simulink library "dali_library"  (Simulink 7.4)
settings: Solver=ode45  StartTime=0.0  StopTime=10.0  RelTol=1e-3
libraries: dali_library x65, xbsIndex_r4 x43, gavrt_library x10, casper_library x1
settings Model: Creator=rprimian  LastModifiedBy=rprimian

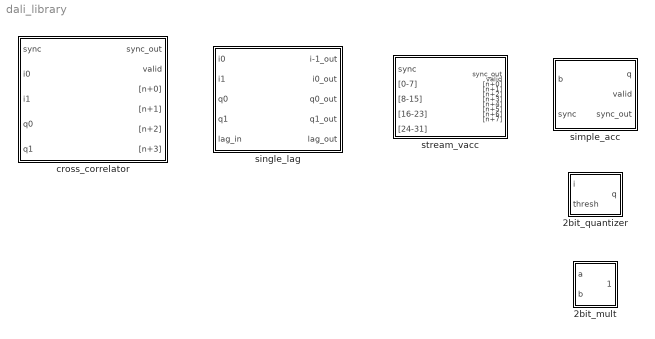
== system dali_library ==
  2bit_mult : Subsystem
      mask Type: 2bit_mult
      mask Description: Implements a special 2-bit multiplier in regular slices. The states represent a symmetric binary encoding where 0, 1, -1, -2 are small-positive, large-positive, small-negative, and large-negative respectively. This is compatible with the 2-bit quantizer
      mask Display:
      | port_label('input', 1, 'a');
      | port_label('input', 2, 'b');
      | port_label('output', 1, '(ab)');
  2bit_quantizer : Subsystem
      mask Type: 2bit_quantizer
      mask Description: Quantizes inputs to a special 2-bit binary encoding using a dynamically set threshold value.
  cross_correlator : Subsystem  mask(cross_correlator){total_lags=5, n_inputs=1, use_2bit=off, input_bit_width=8, input_bin_pt=7, specify_data_type=off, output_bit_width=16, output_bin_pt=14, quantization=Truncate, overflow=Wrap, specify_mult=off, mult_spec=Behavioral, specify_add=off, add_spec=Fabric, mult_delay=3, add_delay=2, single_output=off}
      mask prompts: total_lags "Total Lags Centered at Zero: (2^?)"; n_inputs "Number of Simultaneous Inputs: (2^?)"; use_2bit "Use special 2-bit binary encoding"; input_bit_width "Input Bit Width:"; input_bin_pt "Input Binary Point:"; specify_data_type "Specify output data type"; output_bit_width "Output Bit Width:"; output_bin_pt "Output Binary Point:"; quantization "Quantization Behavior:"; overflow "Overflow Behavior"; specify_mult "Specify multiplier use (behavioural HDL if not specified)"; mult_spec "Multiplier specification:"; specify_add "Specify adder use (behavioural HDL if not specified)"; add_spec "Adder specification:"; mult_delay "Mult Latency:"; add_delay "Add Latency:"; single_output "Provide single output stream"
      mask help: This time-domain cross correlator accepts two real time-series and outputs the cross-correlation function for the given set of lags. The output is accumulated so that for every two input samples there is exactly one output sample.
      mask init:
      | cross_correlator_init(gcb,...
      |     'total_lags', total_lags,...
      |     'n_inputs', n_inputs,...
      |     'use_2bit', use_2bit,...
      |     'input_bit_width', input_bit_width,...
      |     'input_bin_pt', input_bin_pt,...
      |     'specify_data_type', specify_data_type,...
      |     'output_bit_width', output_bit_width,...
      |     'output_bin_pt', output_bin_pt,...
      |     'quantization', quantization,...
      |     'overflow', overflow,...
      |     'specify_mult', specify_mult,...
      |     'mult_spec', mult_spec,...
      |     'specify_add', specify_add,...
      |     'add_spec', add_spec,...
      |     'mult_delay', mult_delay,...
      |     'add_delay', add_delay,...
      |     'single_output', single_output);
      settings: AttributesFormatString=|
      | 32 lags, Demux: 2, Outputs: 4
      | 8_7=>16_14, Truncate, Wrap
      |  Mult: Behavioral, Add: Fabric
      mask StyleString: edit,edit,checkbox,edit,edit,checkbox,edit,edit,popup(Truncate|Round (unbiased: +/- Inf)|Round (unbiased: Even Values)),popup(Wrap|Saturate|Flag as error),checkbox,popup(Behavioral|Core|Embedded),checkbox,popup(Fabric|DSP48),edit,edit,checkbox
      mask CallbackString:
      | ||use_2bit = get_param(gcb,'use_2bit');
      | enables = get_param(gcb, 'MaskEnables');
      | if( strcmp(use_2bit,'on')),
      |     enables{4} = 'off';
      |     enables{5} = 'off';
      | else
      |     enables{4} = 'on';
      |     enables{5} = 'on';
      | end
      | set_param(gcb, 'MaskEnables', enables);
      | |||specify_data_type = get_param(gcb,'specify_data_type');
      | enables = get_param(gcb, 'MaskEnables');
      | if( strcmp(specify_data_type,'off')),
      |     enables{7} = 'off';
      |     enables{8} = 'off';
      |     enables{9} = 'off';
      |     enables{10} = 'off';
      | else
      |     enables{7} = 'on';
      |     enables{8} = 'on';
      |     enables{9} = 'on';
      |     enables{10} = 'on';
      | end
      | set_param(gcb, 'MaskEnables', enables);
      | |||||specify_mult = get_param(gcb,'specify_mult');
      | enables = get_param(gcb, 'MaskEnables');
      | if( strcmp(specify_mult,'off')),
      |     enables{12} = 'off';
      | else
      |     enables{12} = 'on';
      | end
      | set_param(gcb, 'MaskEnables', enables);
      | ||specify_add = get_param(gcb,'specify_add');
      | enables = get_param(gcb, 'MaskEnables');
      | if( strcmp(specify_add,'off')),
      |     enables{14} = 'off';
      | else
      |     enables{14} = 'on';
      | end
      | set_param(gcb, 'MaskEnables', enables);
      | ||||
      mask TabNameString: Basic,Basic,Input,Input,Input,Output,Output,Output,Output,Output,Implementation,Implementation,Implementation,Implementation,Implementation,Implementation,Basic
  simple_acc : Subsystem  mask(simple_acc){samples=2, bit_width=16, bin_pt=14, quantization=Truncate, overflow=Flag as error, specify_add=off, add_spec=Fabric}
      mask prompts: samples "Samples to Accumulate: (2^?)"; bit_width "Output Bit Width:"; bin_pt "Output Binary Point:"; quantization "Quantization Behavior:"; overflow "Overflow Behavior:"; specify_add "Specify adder use (behavioural HDL if not specified)"; add_spec "Adder Specification:"
      mask help: This block accumulates a single stream of data for 2^n samples at a time. The partial sums are full every 2^n clocks and are synced to the falling edge of the sync_out port.
      mask init:
      | set_param([gcb, '/AddSub'], 'Quantization', quantization);
      | set_param([gcb, '/AddSub'], 'Overflow', overflow);
      | if strcmp(specify_add, 'on')
      |     set_param([gcb, '/AddSub'], 'Use_Behavioral_HDL', 'off');
      | else
      |     set_param([gcb, '/AddSub'], 'Use_Behavioral_HDL', 'on');
      | end
      | set_param([gcb, '/AddSub'], 'HW_selection', add_spec);
      mask StyleString: edit,edit,edit,popup(Truncate|Round  (unbiased: +/- Inf)),popup(Wrap|Saturate|Flag as error),checkbox,popup(Fabric|DSP48)
      mask CallbackString:
      | |||||specify_add = get_param(gcb,'specify_add');
      | visibs = get_param(gcb, 'MaskVisibilities');
      | if( strcmp(specify_add,'off')),
      |     visibs{7} = 'off';
      | else
      |     visibs{7} = 'on';
      | end
      | set_param(gcb, 'MaskVisibilities', visibs);|
  single_lag : Subsystem  mask(single_lag){n_inputs=1, specify_mult=off, mult_spec=Behavioral, specify_add=off, add_spec=Fabric, mult_delay=3, add_delay=2, use_2bit=off, shift_q=off, shift_i=on}
      mask prompts: n_inputs "Number of Simultaneous Inputs: (2^?)"; specify_mult "Specify multiplier use (behavioural HDL if not specified)"; mult_spec "Multiplier specification:"; specify_add "Specify adder use (behavioural HDL if not specified)"; add_spec "Adder specification:"; mult_delay "Mult Latency:"; add_delay "Add Latency:"; use_2bit "Use special 2-bit binary encoding"; shift_q "Shift 'q' output"; shift_i "Shift 'i' output"
      mask help: This performs the computations for a single lag. Please use the 'cross_correlator' block to generate a full X-engine.
      mask init:
      | single_lag_init(gcb,...
      |     'n_inputs', n_inputs,...
      |     'specify_mult', specify_mult,...
      |     'mult_spec', mult_spec,...
      |     'specify_add', specify_add,...
      |     'add_spec', add_spec,...
      |     'mult_delay', mult_delay,...
      |     'add_delay', add_delay,...
      |     'use_2bit', use_2bit,...
      |     'shift_q', shift_q,...
      |     'shift_i', shift_i);
      settings: AttributesFormatString=|
      | Use 2-bit: off, Demux: 2,
      | Mult: Behavioral,
      | Add: Fabric
      mask StyleString: edit,checkbox,popup(Behavioral|Core|Embedded),checkbox,popup(Fabric|DSP48),edit,edit,checkbox,checkbox,checkbox
      mask CallbackString:
      | |specify_mult = get_param(gcb,'specify_mult');
      | enables = get_param(gcb, 'MaskEnables');
      | if( strcmp(specify_mult,'off')),
      |     enables{3} = 'off';
      | else,
      |     enables{3} = 'on';
      | end
      | set_param(gcb, 'MaskEnables', enables);
      | ||specify_add = get_param(gcb,'specify_add');
      | enables = get_param(gcb, 'MaskEnables');
      | if( strcmp(specify_add,'off')),
      |     enables{5} = 'off';
      | else,
      |     enables{5} = 'on';
      | end
      | set_param(gcb, 'MaskEnables', enables);
      | ||||||
      mask TabNameString: Basic,Implementation,Implementation,Implementation,Implementation,Implementation,Implementation,Basic,Basic,Basic
  stream_vacc : Subsystem  mask(stream_vacc){vector_len=5, input_bit_width=18, input_bin_pt=14, samples_out=3, output_bit_width=22, output_bin_pt=14, quantization=Truncate, overflow=Wrap, specify_add=off, add_spec=Fabric, add_delay=1}
      mask prompts: vector_len "Vector Length: (2^?)"; input_bit_width "Input Bit Width:"; input_bin_pt "Input Binary Point:"; samples_out "Number of Simultaneous Outputs: (2^?)"; output_bit_width "Output Bit Width:"; output_bin_pt "Output Binary Point:"; quantization "Quantization Behavior:"; overflow "Overflow Behavior:"; specify_add "Specify adder use (behavioural HDL if not specified)"; add_spec "Adder specification:"; add_delay "Add Latency:"
      mask help: This block implements the second stage adder for the cross_correlator block.
      mask init:
      | stream_vacc_init(gcb,...
      |     'vector_len', vector_len,...
      |     'input_bit_width', input_bit_width,...
      |     'input_bin_pt', input_bin_pt,...
      |     'samples_out', samples_out,...
      |     'output_bit_width', output_bit_width,...
      |     'output_bin_pt', output_bin_pt,...
      |     'quantization', quantization,...
      |     'overflow', overflow,...
      |     'specify_add', specify_add,...
      |     'add_spec', add_spec,...
      |     'add_delay', add_delay);
      settings: AttributesFormatString=|
      | 32=>8 samples
      | Accumulate
      mask StyleString: edit,edit,edit,edit,edit,edit,popup(Truncate|Round  (unbiased: +/- Inf)),popup(Wrap|Saturate|Flag as error),checkbox,popup(Fabric|DSP48),edit
      mask CallbackString:
      | |||vector_len = str2num(get_param(gcb, 'vector_len'));
      | samples_out = str2num(get_param(gcb, 'samples_out'));
      | 
      | if vector_len<samples_out,
      |     error('Number of parallel streams must be greater than or equal to the vector length!');
      | end|||||specify_add = get_param(gcb,'specify_add');
      | visibs = get_param(gcb, 'MaskVisibilities');
      | if( strcmp(specify_add,'off')),
      |     visibs{10} = 'off';
      | else
      |     visibs{10} = 'on';
      | end
      | set_param(gcb, 'MaskVisibilities', visibs);||

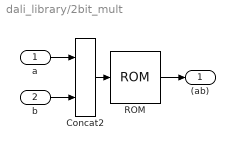
== system dali_library/2bit_mult ==
  a : Inport  OutDataType=sfix(16)  OutScaling=2^0
  b : Inport  Port=2  OutDataType=sfix(16)  OutScaling=2^0
  Concat2 : xbsIndex_r4/Concat  num_inputs=2  dbl_ovrd=off  block_type=concat
      settings: block_version=10.1.3
  ROM : xbsIndex_r4/ROM  depth=16  initVector=[1; 3; -1; -3; 3; 9; -3; -9; -1; -3; 1; 3; -3; -9; 3; 9]  distributed_mem=Distributed memory  rst=off  init_reg=0  en=off  latency=1  arith_type="Signed  (2's comp)"  n_bits=5  bin_pt=0  dbl_ovrd=off  optimize=Area  use_rpm=off  block_type=sprom
      settings: xl_area=[0, 0, 0, 0, 0, 0, 0]  block_version=10.1.3
  (ab) : Outport  OutDataType=sfix(16)  OutScaling=2^0
  wires:
  Concat2/1 -> ROM/1
  a/1 -> Concat2/1
  ROM/1 -> (ab)/1
  b/1 -> Concat2/2

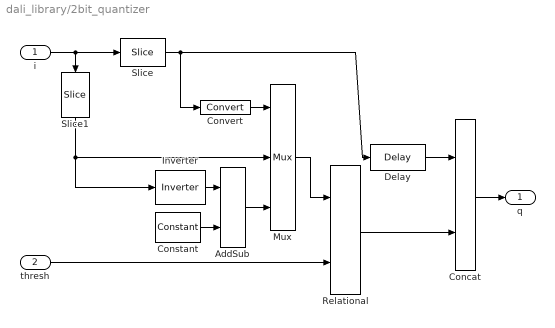
== system dali_library/2bit_quantizer ==
  i : Inport  OutDataType=sfix(16)  OutScaling=2^0
  thresh : Inport  Port=2  OutDataType=sfix(16)  OutScaling=2^0
  AddSub : xbsIndex_r4/AddSub  mode=Addition  use_carryin=off  use_carryout=off  en=off  latency=0  precision=Full  arith_type=Unsigned  n_bits=8  bin_pt=2  quantization=Truncate  overflow=Wrap  dbl_ovrd=off  use_behavioral_HDL=on  hw_selection=Fabric  pipelined=off  use_rpm=on  block_type=addsub
      settings: xl_area=[0, 0, 0, 0, 0, 0, 0]  block_version=10.1.3
  Concat : xbsIndex_r4/Concat  num_inputs=2  dbl_ovrd=off  block_type=concat
      settings: block_version=10.1.3
  Constant : xbsIndex_r4/Constant  arith_type=Unsigned  const=1  n_bits=7  bin_pt=0  explicit_period=on  period=1  equ=P=C  opselect=C  inp2=PCIN>>17  opr=+  inp1=P  carry=CIN  dbl_ovrd=off  block_type=constant
  Convert : xbsIndex_r4/Convert  arith_type=Boolean  n_bits=8  bin_pt=6  quantization=Truncate  overflow=Wrap  latency=0  dbl_ovrd=off  pipeline=off  block_type=convert
      settings: xl_area=[0, 0, 0, 0, 0, 0, 0]  block_version=10.1.3
  Delay : xbsIndex_r4/Delay  en=off  latency=1  dbl_ovrd=off  reg_retiming=off  block_type=delay
      settings: xl_area=[0, 0, 0, 0, 0, 0, 0]
  Inverter : xbsIndex_r4/Inverter  en=off  latency=0  dbl_ovrd=off  block_type=inv
      settings: xl_area=[0, 0, 0, 0, 0, 0, 0]
  Mux : xbsIndex_r4/Mux  inputs=2  en=off  latency=0  precision=Full  arith_type="Signed  (2's comp)"  n_bits=8  bin_pt=2  quantization=Truncate  overflow=Wrap  dbl_ovrd=off  block_type=mux
      settings: xl_area=[0, 0, 0, 0, 0, 0, 0]
  Relational : xbsIndex_r4/Relational  mode=a>=b  en=off  latency=1  dbl_ovrd=off  block_type=relational
      settings: xl_area=[0, 0, 0, 0, 0, 0, 0]  block_version=10.1.3
  Slice : xbsIndex_r4/Slice  nbits=1  boolean_output=off  mode=Upper Bit Location + Width  bit1=0  base1=MSB of Input  bit0=0  base0=LSB of Input  dbl_ovrd=off  block_type=slice
      settings: infoedit="Extracts a given range of bits from each input sample and presents it at the output.  The output type is ordinarily unsigned with binary point at zero, but can be Boolean when the slice is one bit wide.<P><P>Hardware notes: In hardware this block costs nothing."  block_version=10.1.3
  Slice1 : xbsIndex_r4/Slice  nbits=7  boolean_output=off  mode=Upper Bit Location + Width  bit1=-1  base1=MSB of Input  bit0=0  base0=LSB of Input  dbl_ovrd=off  block_type=slice
      settings: infoedit="Extracts a given range of bits from each input sample and presents it at the output.  The output type is ordinarily unsigned with binary point at zero, but can be Boolean when the slice is one bit wide.<P><P>Hardware notes: In hardware this block costs nothing."  block_version=10.1.3
  q : Outport  OutDataType=sfix(16)  OutScaling=2^0
  wires:
  AddSub/1 -> Mux/3
  Slice1/1 -> Inverter/1, Mux/2
  Mux/1 -> Relational/1
  Convert/1 -> Mux/1
  Constant/1 -> AddSub/2
  Inverter/1 -> AddSub/1
  Delay/1 -> Concat/1
  thresh/1 -> Relational/2
  Relational/1 -> Concat/2
  Slice/1 -> Convert/1, Delay/1
  Concat/1 -> q/1
  i/1 -> Slice1/1, Slice/1

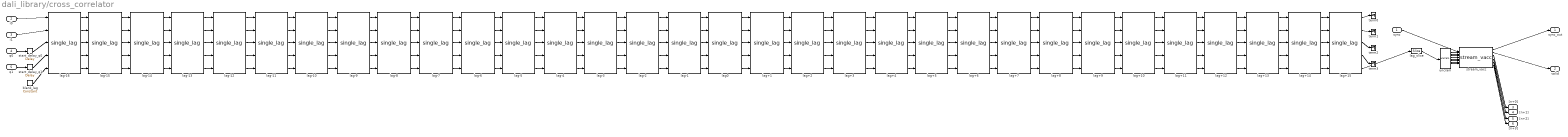
== system dali_library/cross_correlator ==
  sync : Inport
  i0 : Inport  Port=2
  i1 : Inport  Port=3
  q0 : Inport  Port=4
  q1 : Inport  Port=5
  blank_lag : xbsIndex_r4/Constant  arith_type=Unsigned  const=0  n_bits=1  bin_pt=0  explicit_period=on  period=1  equ=P=C  opselect=C  inp2=PCIN>>17  opr=+  inp1=P  carry=CIN  dbl_ovrd=off  block_type=constant
      settings: block_version=11.4
  lag+{1..15} (15 alike) : dali_library/single_lag  SystemSampleTime=-1  n_inputs=1  specify_mult=off  mult_spec=Behavioral  specify_add=off  add_spec=Fabric  mult_delay=3  add_delay=2  use_2bit=off  shift_q=off  shift_i=on
      settings: AttributesFormatString=|
      | Use 2-bit: off, Demux: 2,
      | Mult: Behavioral,
      | Add: Fabric
  lag-{1..16} (16 alike) : dali_library/single_lag  SystemSampleTime=-1  n_inputs=1  specify_mult=off  mult_spec=Behavioral  specify_add=off  add_spec=Fabric  mult_delay=3  add_delay=2  use_2bit=off  shift_q=off  shift_i=on
      settings: AttributesFormatString=|
      | Use 2-bit: off, Demux: 2,
      | Mult: Behavioral,
      | Add: Fabric
  lag0 : dali_library/single_lag  SystemSampleTime=-1  n_inputs=1  specify_mult=off  mult_spec=Behavioral  specify_add=off  add_spec=Fabric  mult_delay=3  add_delay=2  use_2bit=off  shift_q=off  shift_i=on
      settings: AttributesFormatString=|
      | Use 2-bit: off, Demux: 2,
      | Mult: Behavioral,
      | Add: Fabric
  lag_slice : xbsIndex_r4/Slice  nbits=544  boolean_output=off  mode=Lower Bit Location + Width  bit1=0  base1=MSB of Input  bit0=0  base0=LSB of Input  dbl_ovrd=off  block_type=slice
  start_delay_q0 : xbsIndex_r4/Delay  en=off  latency=8  dbl_ovrd=off  reg_retiming=off  block_type=delay
      settings: block_version=11.4
  start_delay_q1 : xbsIndex_r4/Delay  en=off  latency=8  dbl_ovrd=off  reg_retiming=off  block_type=delay
      settings: block_version=11.4
  stream_vacc : dali_library/stream_vacc  SystemSampleTime=-1  vector_len=5  input_bit_width=17  input_bin_pt=14  samples_out=2  output_bit_width=25  output_bin_pt=14  quantization=Truncate  overflow=Wrap  specify_add=off  add_spec=Fabric  add_delay=1
      settings: AttributesFormatString=|
      | 32=>4 samples
      | Accumulate
  term{0..3} (4 alike) : Terminator
  uncram : gavrt_library/uncram  SystemSampleTime=-1  num_slice=8  slice_width=68  bin_pt=0  arith_type=0
      settings: AttributesFormatString=UFix_68_0
  sync_out : Outport
  valid : Outport  Port=2
  "[n+0]" : Outport  Port=3
  "[n+1]" : Outport  Port=4
  "[n+2]" : Outport  Port=5
  "[n+3]" : Outport  Port=6
  wires:
  q0/1 -> start_delay_q0/1
  q1/1 -> start_delay_q1/1
  blank_lag/1 -> lag-16/5
  i0/1 -> lag-16/1
  start_delay_q0/1 -> lag-16/3
  i1/1 -> lag-16/2
  start_delay_q1/1 -> lag-16/4
  lag-16/1 -> lag-15/1
  lag-16/2 -> lag-15/2
  lag-16/3 -> lag-15/3
  lag-16/4 -> lag-15/4
  lag-16/5 -> lag-15/5
  lag-15/1 -> lag-14/1
  lag-15/2 -> lag-14/2
  lag-15/3 -> lag-14/3
  lag-15/4 -> lag-14/4
  lag-15/5 -> lag-14/5
  lag-14/1 -> lag-13/1
  lag-14/2 -> lag-13/2
  lag-14/3 -> lag-13/3
  lag-14/4 -> lag-13/4
  lag-14/5 -> lag-13/5
  lag-13/1 -> lag-12/1
  lag-13/2 -> lag-12/2
  lag-13/3 -> lag-12/3
  lag-13/4 -> lag-12/4
  lag-13/5 -> lag-12/5
  lag-12/1 -> lag-11/1
  lag-12/2 -> lag-11/2
  lag-12/3 -> lag-11/3
  lag-12/4 -> lag-11/4
  lag-12/5 -> lag-11/5
  lag-11/1 -> lag-10/1
  lag-11/2 -> lag-10/2
  lag-11/3 -> lag-10/3
  lag-11/4 -> lag-10/4
  lag-11/5 -> lag-10/5
  lag-10/1 -> lag-9/1
  lag-10/2 -> lag-9/2
  lag-10/3 -> lag-9/3
  lag-10/4 -> lag-9/4
  lag-10/5 -> lag-9/5
  lag-9/1 -> lag-8/1
  lag-9/2 -> lag-8/2
  lag-9/3 -> lag-8/3
  lag-9/4 -> lag-8/4
  lag-9/5 -> lag-8/5
  lag-8/1 -> lag-7/1
  lag-8/2 -> lag-7/2
  lag-8/3 -> lag-7/3
  lag-8/4 -> lag-7/4
  lag-8/5 -> lag-7/5
  lag-7/1 -> lag-6/1
  lag-7/2 -> lag-6/2
  lag-7/3 -> lag-6/3
  lag-7/4 -> lag-6/4
  lag-7/5 -> lag-6/5
  lag-6/1 -> lag-5/1
  lag-6/2 -> lag-5/2
  lag-6/3 -> lag-5/3
  lag-6/4 -> lag-5/4
  lag-6/5 -> lag-5/5
  lag-5/1 -> lag-4/1
  lag-5/2 -> lag-4/2
  lag-5/3 -> lag-4/3
  lag-5/4 -> lag-4/4
  lag-5/5 -> lag-4/5
  lag-4/1 -> lag-3/1
  lag-4/2 -> lag-3/2
  lag-4/3 -> lag-3/3
  lag-4/4 -> lag-3/4
  lag-4/5 -> lag-3/5
  lag-3/1 -> lag-2/1
  lag-3/2 -> lag-2/2
  lag-3/3 -> lag-2/3
  lag-3/4 -> lag-2/4
  lag-3/5 -> lag-2/5
  lag-2/1 -> lag-1/1
  lag-2/2 -> lag-1/2
  lag-2/3 -> lag-1/3
  lag-2/4 -> lag-1/4
  lag-2/5 -> lag-1/5
  lag-1/1 -> lag0/1
  lag-1/2 -> lag0/2
  lag-1/3 -> lag0/3
  lag-1/4 -> lag0/4
  lag-1/5 -> lag0/5
  lag0/1 -> lag+1/1
  lag0/2 -> lag+1/2
  lag0/3 -> lag+1/3
  lag0/4 -> lag+1/4
  lag0/5 -> lag+1/5
  lag+1/1 -> lag+2/1
  lag+1/2 -> lag+2/2
  lag+1/3 -> lag+2/3
  lag+1/4 -> lag+2/4
  lag+1/5 -> lag+2/5
  lag+2/1 -> lag+3/1
  lag+2/2 -> lag+3/2
  lag+2/3 -> lag+3/3
  lag+2/4 -> lag+3/4
  lag+2/5 -> lag+3/5
  lag+3/1 -> lag+4/1
  lag+3/2 -> lag+4/2
  lag+3/3 -> lag+4/3
  lag+3/4 -> lag+4/4
  lag+3/5 -> lag+4/5
  lag+4/1 -> lag+5/1
  lag+4/2 -> lag+5/2
  lag+4/3 -> lag+5/3
  lag+4/4 -> lag+5/4
  lag+4/5 -> lag+5/5
  lag+5/1 -> lag+6/1
  lag+5/2 -> lag+6/2
  lag+5/3 -> lag+6/3
  lag+5/4 -> lag+6/4
  lag+5/5 -> lag+6/5
  lag+6/1 -> lag+7/1
  lag+6/2 -> lag+7/2
  lag+6/3 -> lag+7/3
  lag+6/4 -> lag+7/4
  lag+6/5 -> lag+7/5
  lag+7/1 -> lag+8/1
  lag+7/2 -> lag+8/2
  lag+7/3 -> lag+8/3
  lag+7/4 -> lag+8/4
  lag+7/5 -> lag+8/5
  lag+8/1 -> lag+9/1
  lag+8/2 -> lag+9/2
  lag+8/3 -> lag+9/3
  lag+8/4 -> lag+9/4
  lag+8/5 -> lag+9/5
  lag+9/1 -> lag+10/1
  lag+9/2 -> lag+10/2
  lag+9/3 -> lag+10/3
  lag+9/4 -> lag+10/4
  lag+9/5 -> lag+10/5
  lag+10/1 -> lag+11/1
  lag+10/2 -> lag+11/2
  lag+10/3 -> lag+11/3
  lag+10/4 -> lag+11/4
  lag+10/5 -> lag+11/5
  lag+11/1 -> lag+12/1
  lag+11/2 -> lag+12/2
  lag+11/3 -> lag+12/3
  lag+11/4 -> lag+12/4
  lag+11/5 -> lag+12/5
  lag+12/1 -> lag+13/1
  lag+12/2 -> lag+13/2
  lag+12/3 -> lag+13/3
  lag+12/4 -> lag+13/4
  lag+12/5 -> lag+13/5
  lag+13/1 -> lag+14/1
  lag+13/2 -> lag+14/2
  lag+13/3 -> lag+14/3
  lag+13/4 -> lag+14/4
  lag+13/5 -> lag+14/5
  lag+14/1 -> lag+15/1
  lag+14/2 -> lag+15/2
  lag+14/3 -> lag+15/3
  lag+14/4 -> lag+15/4
  lag+14/5 -> lag+15/5
  lag+15/1 -> term0/1
  lag+15/2 -> term1/1
  lag+15/3 -> term2/1
  lag+15/4 -> term3/1
  lag+15/5 -> lag_slice/1
  lag_slice/1 -> uncram/1
  sync/1 -> stream_vacc/1
  uncram/1 -> stream_vacc/2
  uncram/2 -> stream_vacc/3
  uncram/3 -> stream_vacc/4
  uncram/4 -> stream_vacc/5
  uncram/5 -> stream_vacc/6
  uncram/6 -> stream_vacc/7
  uncram/7 -> stream_vacc/8
  uncram/8 -> stream_vacc/9
  stream_vacc/1 -> sync_out/1
  stream_vacc/2 -> valid/1
  stream_vacc/3 -> "[n+0]"/1
  stream_vacc/4 -> "[n+1]"/1
  stream_vacc/5 -> "[n+2]"/1
  stream_vacc/6 -> "[n+3]"/1

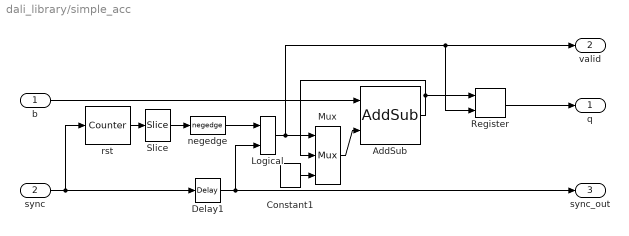
== system dali_library/simple_acc ==
  b : Inport
  sync : Inport  Port=2
  AddSub : xbsIndex_r4/AddSub  mode=Addition  use_carryin=off  use_carryout=off  en=off  latency=1  precision=User Defined  arith_type="Signed  (2's comp)"  n_bits=bit_width  bin_pt=bin_pt  quantization=Truncate  overflow=Flag as error  dbl_ovrd=off  use_behavioral_HDL=on  hw_selection=Fabric  pipelined=off  block_type=addsub
      settings: block_version=11.3
  Constant1 : xbsIndex_r4/Constant  arith_type=Signed (2's comp)  const=0  n_bits=bit_width  bin_pt=bin_pt  explicit_period=on  period=1  equ=P=C  opselect=C  inp2=PCIN>>17  opr=+  inp1=P  carry=CIN  dbl_ovrd=off  block_type=constant
      settings: block_version=11.3
  Delay1 : xbsIndex_r4/Delay  en=off  latency=1  dbl_ovrd=off  reg_retiming=off  block_type=delay
      settings: block_version=11.3
  Logical : xbsIndex_r4/Logical  logical_function=OR  inputs=2  en=off  latency=0  precision=Full  arith_type=Unsigned  n_bits=16  bin_pt=0  align_bp=on  dbl_ovrd=off  block_type=logical
      settings: block_version=11.3
  Mux : xbsIndex_r4/Mux  inputs=2  en=off  latency=0  precision=Full  arith_type=Unsigned  n_bits=16  bin_pt=14  quantization=Truncate  overflow=Wrap  dbl_ovrd=off  block_type=mux
      settings: block_version=11.3
  Register : xbsIndex_r4/Register  init=0  rst=off  en=on  dbl_ovrd=off  block_type=register
      settings: block_version=11.3
  Slice : xbsIndex_r4/Slice  nbits=1  boolean_output=on  mode=Upper Bit Location + Width  bit1=0  base1=MSB of Input  bit0=0  base0=LSB of Input  dbl_ovrd=off  block_type=slice
      settings: block_version=11.3
  negedge : casper_library/Misc/negedge  Tag=Rising Edge Detector  SystemSampleTime=-1
  rst : xbsIndex_r4/Counter  cnt_type=Free Running  cnt_to=Inf  operation=Up  start_count=0  cnt_by_val=1  arith_type=Unsigned  n_bits=samples  bin_pt=0  load_pin=off  rst=on  en=off  explicit_period=on  period=1  dbl_ovrd=off  use_behavioral_HDL=off  implementation=Fabric  block_type=counter
      settings: block_version=11.3
  q : Outport
  valid : Outport  Port=2
  sync_out : Outport  Port=3
  wires:
  Register/1 -> q/1
  Delay1/1 -> Logical/2, sync_out/1
  negedge/1 -> Logical/1
  Logical/1 -> Mux/1, Register/2, valid/1
  Slice/1 -> negedge/1
  rst/1 -> Slice/1
  sync/1 -> Delay1/1, rst/1
  b/1 -> AddSub/1
  Constant1/1 -> Mux/3
  AddSub/1 -> Mux/2, Register/1
  Mux/1 -> AddSub/2

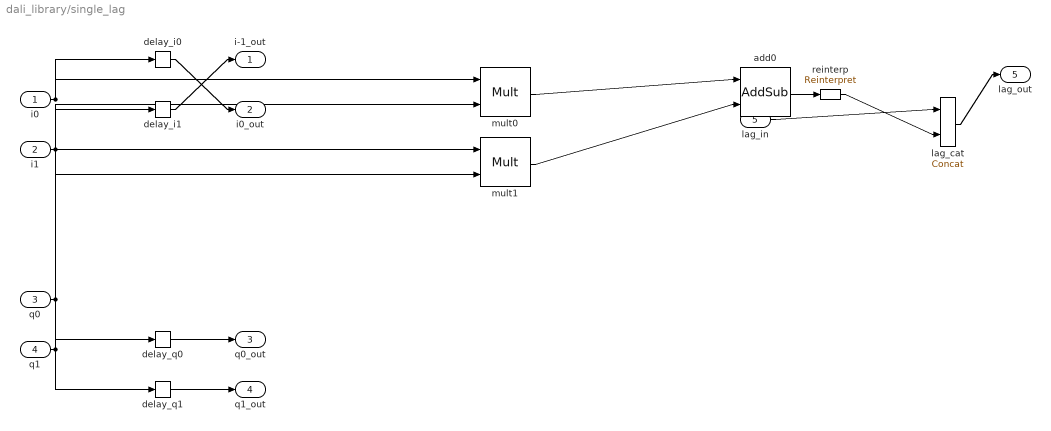
== system dali_library/single_lag ==
  i0 : Inport
  i1 : Inport  Port=2
  q0 : Inport  Port=3
  q1 : Inport  Port=4
  lag_in : Inport  Port=5
  add0 : xbsIndex_r4/AddSub  mode=Addition  use_carryin=off  use_carryout=off  en=off  latency=2  precision=Full  arith_type=Unsigned  n_bits=16  bin_pt=14  quantization=Truncate  overflow=Wrap  dbl_ovrd=off  use_behavioral_HDL=on  hw_selection=Fabric  pipelined=on  block_type=addsub
  delay_i0 : xbsIndex_r4/Delay  en=off  latency=0  dbl_ovrd=off  reg_retiming=off  block_type=delay
      settings: block_version=11.4
  delay_i1 : xbsIndex_r4/Delay  en=off  latency=1  dbl_ovrd=off  reg_retiming=off  block_type=delay
      settings: block_version=11.4
  delay_q0 : xbsIndex_r4/Delay  en=off  latency=0  dbl_ovrd=off  reg_retiming=off  block_type=delay
      settings: block_version=11.4
  delay_q1 : xbsIndex_r4/Delay  en=off  latency=0  dbl_ovrd=off  reg_retiming=off  block_type=delay
      settings: block_version=11.4
  lag_cat : xbsIndex_r4/Concat  num_inputs=2  dbl_ovrd=off  block_type=concat
  mult0 : xbsIndex_r4/Mult  precision=Full  arith_type="Signed  (2's comp)"  n_bits=16  bin_pt=14  quantization=Truncate  overflow=Wrap  en=off  latency=3  dbl_ovrd=off  use_behavioral_HDL=on  opt=Speed  use_embedded=off  optimum_pipeline=off  pipeline=on  use_rpm=on  placement_style=Triangular  block_type=mult
      settings: block_version=11.4
  mult1 : xbsIndex_r4/Mult  precision=Full  arith_type="Signed  (2's comp)"  n_bits=16  bin_pt=14  quantization=Truncate  overflow=Wrap  en=off  latency=3  dbl_ovrd=off  use_behavioral_HDL=on  opt=Speed  use_embedded=off  optimum_pipeline=off  pipeline=on  use_rpm=on  placement_style=Triangular  block_type=mult
      settings: block_version=11.4
  reinterp : xbsIndex_r4/Reinterpret  force_arith_type=on  arith_type=Unsigned  force_bin_pt=on  bin_pt=0  block_type=reinterpret
      settings: infoedit="Changes signal type without altering the binary representation.   You can changed the signal between signed and unsigned, and relocate the binary point.<br><br>Hardware notes: In hardware this block costs nothing.<br><br>Example:  Suppose the input is 6 bits wide, signed, with 2 fractional bits, and the output is forced to unsigned with 0 fractional bits.  Then an input of -2.0 (1110.00 in binary 2's complement) becomes an output of 56 (111000 in binary)."
  i-1_out : Outport
  i0_out : Outport  Port=2
  q0_out : Outport  Port=3
  q1_out : Outport  Port=4
  lag_out : Outport  Port=5
  wires:
  i0/1 -> mult0/1, delay_i0/1
  q0/1 -> mult0/2, delay_q0/1
  i1/1 -> mult1/1, delay_i1/1
  q1/1 -> mult1/2, delay_q1/1
  mult0/1 -> add0/1
  mult1/1 -> add0/2
  delay_i0/1 -> i0_out/1
  delay_q0/1 -> q0_out/1
  delay_i1/1 -> i-1_out/1
  delay_q1/1 -> q1_out/1
  lag_in/1 -> lag_cat/1
  add0/1 -> reinterp/1
  reinterp/1 -> lag_cat/2
  lag_cat/1 -> lag_out/1

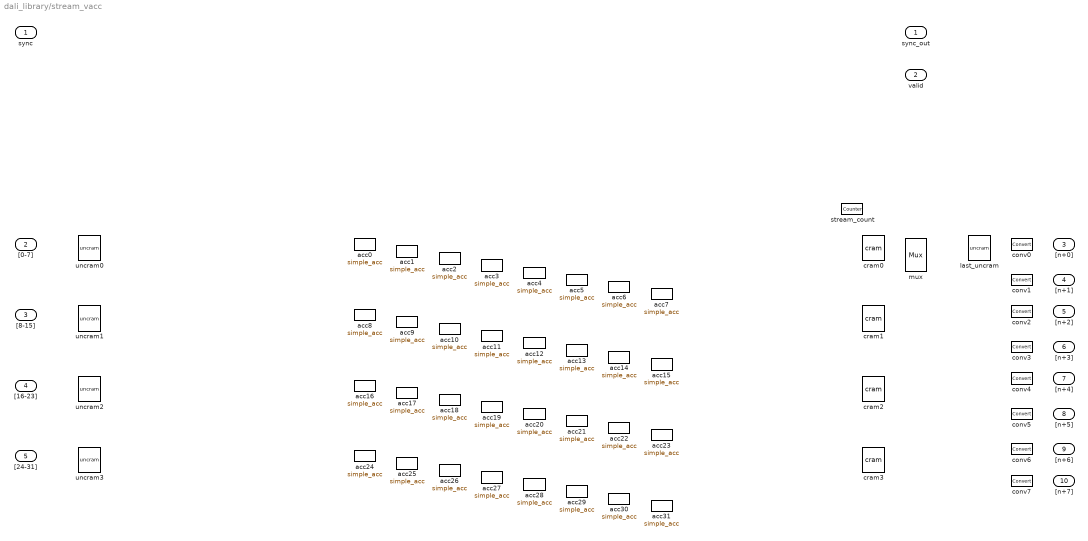
== system dali_library/stream_vacc ==
  sync : Inport
  "[0-7]" : Inport  Port=2
  "[8-15]" : Inport  Port=3
  "[16-23]" : Inport  Port=4
  "[24-31]" : Inport  Port=5
  acc{0..31} (32 alike) : dali_library/simple_acc  SystemSampleTime=-1  samples=2  bit_width=22  bin_pt=14  quantization=Truncate  overflow=Wrap  specify_add=off  add_spec=Fabric
  conv{0..7} (8 alike) : xbsIndex_r4/Convert  arith_type="Signed  (2's comp)"  n_bits=22  bin_pt=14  quantization=Truncate  overflow=Wrap  latency=0  dbl_ovrd=off  pipeline=off  block_type=convert
      settings: block_version=11.4
  cram{0..3} (4 alike) : gavrt_library/cram  SystemSampleTime=-1  num_slice=8
  last_uncram : gavrt_library/uncram  SystemSampleTime=-1  num_slice=8  slice_width=22  bin_pt=14  arith_type=1
      settings: AttributesFormatString=Fix_22_14
  mux : xbsIndex_r4/Mux  inputs=4  en=off  latency=0  precision=Full  arith_type=Unsigned  n_bits=16  bin_pt=14  quantization=Truncate  overflow=Wrap  dbl_ovrd=off  block_type=mux
      settings: block_version=11.4
  stream_count : xbsIndex_r4/Counter  cnt_type=Free Running  cnt_to=Inf  operation=Up  start_count=0  cnt_by_val=1  arith_type=Unsigned  n_bits=-1  bin_pt=0  load_pin=off  rst=on  en=off  explicit_period=on  period=1  dbl_ovrd=off  use_behavioral_HDL=off  implementation=Fabric  block_type=counter
      settings: block_version=11.4
  uncram{0..3} (4 alike) : gavrt_library/uncram  SystemSampleTime=-1  num_slice=8  slice_width=18  bin_pt=14  arith_type=1
      settings: AttributesFormatString=Fix_18_14
  sync_out : Outport
  valid : Outport  Port=2
  "[n+0]" : Outport  Port=3
  "[n+1]" : Outport  Port=4
  "[n+2]" : Outport  Port=5
  "[n+3]" : Outport  Port=6
  "[n+4]" : Outport  Port=7
  "[n+5]" : Outport  Port=8
  "[n+6]" : Outport  Port=9
  "[n+7]" : Outport  Port=10
